simulink model "LAB5T1"  (R2018b)
settings: Solver=ode113  StartTime=0.0  StopTime=100  RelTol=1e-5  EnableMultiTasking=on
settings Model: Creator=jsb12221  LastModifiedBy=aloisia
settings DataIOCC: LimitDataPoints=on  SaveFormat=Array  SignalLoggingSaveFormat=ModelDataLogs
settings OptimizationCC: ExpressionDepthLimit=2147483647  LifeSpan=inf
settings DebuggingCC: UnderspecifiedInitializationDetection=Classic  MergeDetectMultiDrivingBlocksExec=none  FcnCallInpInsideContextMsg=warning  UnknownTsInhSupMsg=none  StateNameClashWarn=warning  LibraryContextMissingDiagnostic=none  SFUnexpectedBacktrackingDiag=warning  SFNoUnconditionalDefaultTransitionDiag=warning  SFExecutionAtInitializationDiag=none
settings HardwareCC: ProdBitPerPointer=32  ProdBitPerSizeT=32  ProdBitPerPtrDiffT=32  ProdLargestAtomicFloat=None  ProdIntDivRoundTo=Undefined  ProdEndianess=Unspecified  ProdWordSize=32  ProdHWDeviceType=32-bit Generic
settings ModelReferenceCC: PropagateSignalLabelsOutOfModel=off
settings SFSimCC: SimUseLocalCustomCode=off
settings RTWCC: RTWUseLocalCustomCode=off
settings CodeAppCC: StateflowObjectComments=on
settings GRTTargetCC: TargetLangStandard=C89/C90 (ANSI)  GeneratePreprocessorConditionals=Disable all
settings ConfigComp: CovMetricSettings=dw  CovHtmlReporting=on  CovSaveCumulativeToWorkspaceVar=on  CovSaveSingleToWorkspaceVar=on  CovExternalEMLEnable=off

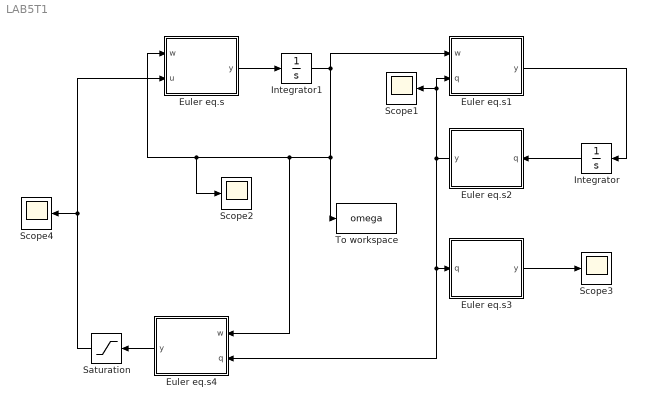
== system LAB5T1 ==
  Euler eq.s : MATLAB Function  TreatAsAtomicUnit=on
  Euler eq.s1 : MATLAB Function  TreatAsAtomicUnit=on
  Euler eq.s2 : MATLAB Function  TreatAsAtomicUnit=on
  Euler eq.s3 : MATLAB Function  TreatAsAtomicUnit=on
  Euler eq.s4 : MATLAB Function  TreatAsAtomicUnit=on
  Integrator : Integrator  InitialCondition=[0.233; -0.667; 0.667; 0.233]
  Integrator1 : Integrator  InitialCondition=[0; 0; 0]
  Saturation : Saturate  UpperLimit=1e-3  LowerLimit=-1e-3
  Scope{1..4} (4 alike) : Scope
  To workspace : ToWorkspace  VariableName=omega  SampleTime=-1
  wires:
  Integrator1/1 -> Euler eq.s1/1(w), To workspace/1, Euler eq.s4/1(w), Scope2/1, Euler eq.s/1(w)
  Euler eq.s/1(y) -> Integrator1/1
  Euler eq.s1/1(y) -> Integrator/1
  Integrator/1 -> Euler eq.s2/1(q)
  Euler eq.s2/1(y) -> Euler eq.s4/2(q), Euler eq.s3/1(q), Scope1/1, Euler eq.s1/2(q)
  Euler eq.s3/1(y) -> Scope3/1
  Euler eq.s4/1(y) -> Saturation/1
  Saturation/1 -> Scope4/1, Euler eq.s/2(u)

== matlab function LAB5T1/Euler eq.s1 ==
  data: w input; y output; q input
function y = quaternion(w,q)


OM = [0 w(3) -w(2) w(1); -w(3) 0 w(1) w(2);...
      w(2) -w(1) 0 w(3); -w(1) -w(2) -w(3) 0];
  
qdot = 0.5.*OM*q;

y=qdot;

== matlab function LAB5T1/Euler eq.s2 ==
  data: y output; q input
function y = norm_quaternion(q)


q = q/norm(q);

y=q;

== matlab function LAB5T1/Euler eq.s3 ==
  data: y output; q input
function y = attitude_q(q)

q1 = q(1);
q2 = q(2);
q3 = q(3);
q4 = q(4);

A = [q1^2-q2^2-q3^2+q4^2 2*(q1*q2+q3*q4) 2*(q1*q3-q2*q4);...
    2*(q1*q2-q3*q4) -q1^2+q2^2-q3^2+q4^2 2*(q2*q3+q1*q4);...
    2*(q1*q3+q2*q4) 2*(q2*q3-q1*q4) -q1^2-q2^2+q3^2+q4^2];

theta = zeros(3,1);
theta(1) = acos(A(3,3));
theta(2) = -atan(A(3,1)/A(3,2));
theta(3) = atan(A(1,3)/A(2,3));

% theta(1) = asin(A(3,1));
% theta(2) = -atan(A(3,2)/A(3,3));
% theta(3) = -atan(A(1,2)/A(1,1));


y=theta;

== matlab function LAB5T1/Euler eq.s ==
  data: w input; y output; u input
function y = euler_eqs(w,u)

J1=0.01;
J2=0.05;
J3=0.07;

w_dot = zeros(3,1);

c1 = ((J2-J3)/J1);
c2 = ((J3-J1)/J2);
c3 = ((J1-J2)/J3);

w_dot(1) = c1*w(2)*w(3) + u(1)/J1;
w_dot(2) = c2*w(1)*w(3) + u(2)/J2;
w_dot(3) = c3*w(2)*w(1) + u(3)/J3;

y=w_dot;

== matlab function LAB5T1/Euler eq.s4 ==
  data: w input; y output; q input
function y = control_law(w,q)

J1=0.01;
J2=0.05;
J3=0.07;

J = diag([J1,J2,J3]);

% Set k1 and k2 due to have a faster stabilization
k1 = 0.5;
k2 = 0.5;

K = k1 * J;
C = k2 * J;

% Change dimension of q

q = [q(1), q(2), q(3)]';
u = -K*q -C*w;

y=u;
